simulink model "explomodel"  (R2017b)
settings: Solver=VariableStepAuto  StartTime=0.0  StopTime=.2  MaxStep=1e-4  RelTol=1e-3
libraries: powerlib x11
settings Model: Creator=K  LastModifiedBy=K

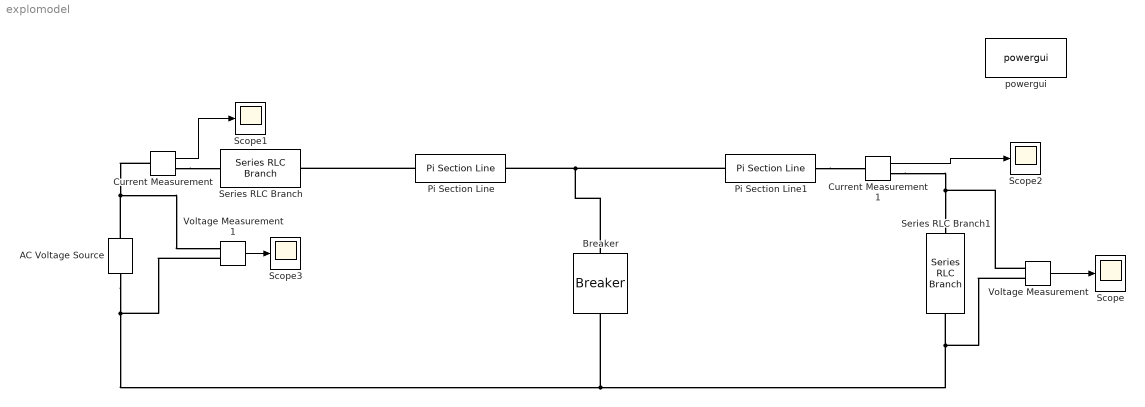
== system explomodel ==
  AC Voltage Source : powerlib/Electrical Sources/AC Voltage Source  Amplitude=220000  Phase=0  Frequency=50  SampleTime=0  Measurements=None  BusType=swing  Pref=10e3  Qref=0  Qmin=-inf  Qmax=+inf
  Breaker : powerlib/Elements/Breaker  InitialState=0  SwitchingTimes="[.1  .15]"  External=off  BreakerResistance=0  SnubberResistance=1e6  SnubberCapacitance=inf  Measurements=None  MoreParameters=on  NoBreakLoop=off
      settings: SourceProductName=Simscape Power Systems
  Current Measurement : powerlib/Measurements/Current Measurement  PhasorSimulation=off  OutputType=Complex  PSBequivalent=0
  Current Measurement1 : powerlib/Measurements/Current Measurement  PhasorSimulation=off  OutputType=Complex  PSBequivalent=0
  Pi Section Line : powerlib/Elements/Pi Section Line  LConnTagsString=__new0  RConnTagsString=__new0  Frequency=50  Resistance=0.01273  Inductance=0.9337e-3  Capacitance=12.74e-9  Length=150  PiSections=1  Measurements=None
      settings: AttributesFormatString=\n  SourceProductName=Simscape Power Systems  SourceProductBaseCode=PS
  Pi Section Line1 : powerlib/Elements/Pi Section Line  LConnTagsString=__new0  RConnTagsString=__new0  Frequency=50  Resistance=0.01273  Inductance=0.9337e-3  Capacitance=12.74e-9  Length=50  PiSections=1  Measurements=None
      settings: AttributesFormatString=\n  SourceProductName=Simscape Power Systems  SourceProductBaseCode=PS
  Scope{,1..3} (4 alike) : Scope
  Series RLC Branch : powerlib/Elements/Series RLC Branch  LConnTagsString=__new0  RConnTagsString=__new0  BranchType=RL  Resistance=1  Inductance=1e-3  SetiL0=off  InitialCurrent=0  Capacitance=1e-6  Setx0=off  InitialVoltage=0  Measurements=None
  Series RLC Branch1 : powerlib/Elements/Series RLC Branch  LConnTagsString=__new0  RConnTagsString=__new0  BranchType=R  Resistance=1  Inductance=1e-3  SetiL0=off  InitialCurrent=0  Capacitance=1e-6  Setx0=off  InitialVoltage=0  Measurements=None
  Voltage Measurement : powerlib/Measurements/Voltage Measurement  PhasorSimulation=off  OutputType=Complex  PSBequivalent=0
  Voltage Measurement1 : powerlib/Measurements/Voltage Measurement  PhasorSimulation=off  OutputType=Complex  PSBequivalent=0
  powergui : powerlib/powergui  Priority=1  SimulationMode=Continuous  SampleTime=50e-6  frequency=60  Iterations=50  frequencyindice=50  Pbase=100e6  ErrMax=1e-4  UnitsV=kV  UnitsW=MW  buscounter=0  FunctionMessages=off  echomessages=off  EnableUseOfTLC=off  CurrentSourceSwitches=off  DisableSnubberDevices=off  DisableRonSwitches=off  DisableVfSwitches=off  DisplayEquations=off  SolverType=Tustin/Backward Euler (TBE)  Interpol=off  ExternalGateDelay=off  methode=off  Ts=100  x0status=blocks  SPID=on  SwTol=0  HookPort=off  RestoreLinks=warning  ResistiveCurrentMeasurement=off  Frange=[0:2:500]  Ylog=off  Xlog=on  ShowGrid=off  save=off  variable=ZData  structure=0  ZoomFFT=off  StartTime=0.0  cycles=1  DisplayStyle=1  fundamental=60  FreqAxis=off  MaxFrequency=1000  frequencyindicesteady=1  RmsSteady=1  display=off
  wires:
  Voltage Measurement/1 -> Scope/1
  Current Measurement/1 -> Scope1/1
  Voltage Measurement1/1 -> Scope3/1
  Current Measurement1/1 -> Scope2/1
  connections:
  Pi Section Line/LConn1 -- Series RLC Branch/RConn1
  Pi Section Line1/LConn1 -- Breaker/LConn1 -- Pi Section Line/RConn1
  AC Voltage Source/RConn1 -- Current Measurement/LConn1 -- Voltage Measurement1/LConn1
  Voltage Measurement/LConn1 -- Series RLC Branch1/LConn1 -- Current Measurement1/RConn1
  AC Voltage Source/LConn1 -- Voltage Measurement1/LConn2 -- Breaker/RConn1 -- Voltage Measurement/LConn2 -- Series RLC Branch1/RConn1
  Current Measurement/RConn1 -- Series RLC Branch/LConn1
  Pi Section Line1/RConn1 -- Current Measurement1/LConn1
